simulink model "MineModel"  (R2024b)
settings: Solver=FixedStepAuto  StartTime=0.0  StopTime=5  FixedStep=1  RelTol=1e-3
values from neighbouring files (symbols this model uses):
  discountRate = dataFixed(4)    [practicalassignment.m]
undefined symbols (not defined in the file or in its folder): initialMiningCost, miningCostInflationRate
settings Model: Creator=veeti  LastModifiedBy=veeti

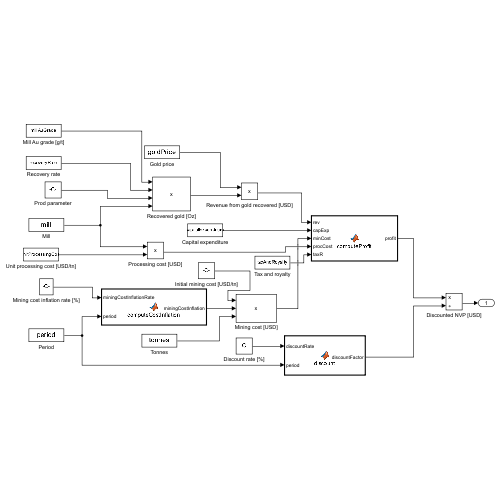
[thumbnail: Simulink's stored preview of the top-level diagram]
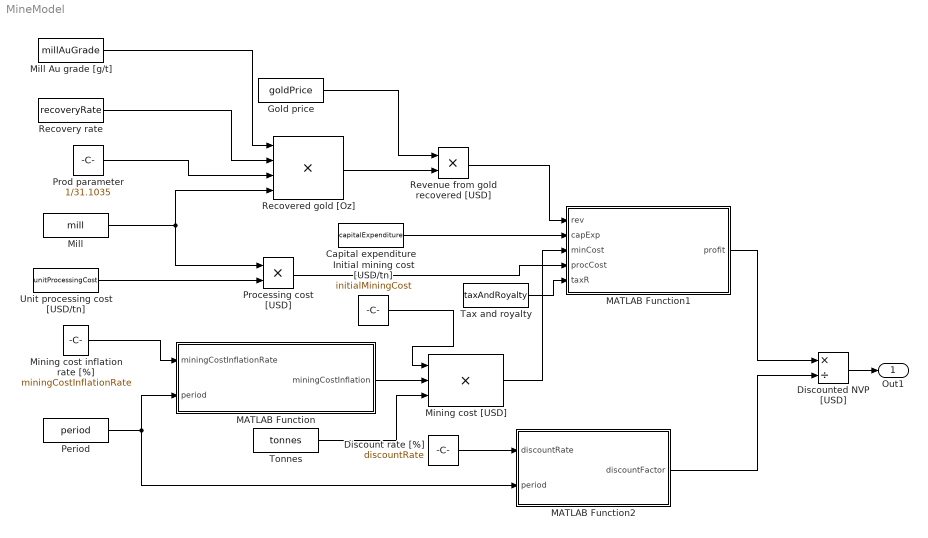
== system MineModel ==
  Capital expenditure : FromWorkspace  VariableName=capitalExpenditure
  Discount rate [%] : Constant  Value=discountRate
  Discounted NVP [USD] : Product  Inputs=*/
  Gold price : FromWorkspace  VariableName=goldPrice
  Initial mining cost [USD/tn] : Constant  Value=initialMiningCost
  MATLAB Function : MATLAB Function  TreatAsAtomicUnit=on
  MATLAB Function1 : MATLAB Function  TreatAsAtomicUnit=on
  MATLAB Function2 : MATLAB Function  TreatAsAtomicUnit=on
  Mill : FromWorkspace  VariableName=mill
  Mill Au grade [g/t] : FromWorkspace  VariableName=millAuGrade
  Mining cost [USD] : Product  Inputs=3
  Mining cost inflation rate [%] : Constant  Value=miningCostInflationRate
  Period : FromWorkspace  VariableName=period
  Processing cost [USD] : Product
  Prod parameter : Constant  Value=1/31.1035
  Recovered gold [Oz] : Product  Inputs=4
  Recovery rate : FromWorkspace  VariableName=recoveryRate
  Revenue from gold recovered [USD] : Product
  Tax and royalty : FromWorkspace  VariableName=taxAndRoyalty
  Tonnes : FromWorkspace  VariableName=tonnes
  Unit processing cost [USD/tn] : FromWorkspace  VariableName=unitProcessingCost
  Out1 : Outport
  wires:
  Mill/1 -> Recovered gold [Oz]/4, Processing cost [USD]/1
  Mill Au grade [g/t]/1 -> Recovered gold [Oz]/1
  Recovery rate/1 -> Recovered gold [Oz]/2
  Prod parameter/1 -> Recovered gold [Oz]/3
  Unit processing cost [USD/tn]/1 -> Processing cost [USD]/2
  Period/1 -> MATLAB Function2/2(period), MATLAB Function/2(period)
  Initial mining cost [USD/tn]/1 -> Mining cost [USD]/1
  MATLAB Function/1(miningCostInflation) -> Mining cost [USD]/2
  Tonnes/1 -> Mining cost [USD]/3
  Recovered gold [Oz]/1 -> Revenue from gold recovered [USD]/2
  Gold price/1 -> Revenue from gold recovered [USD]/1
  Revenue from gold recovered [USD]/1 -> MATLAB Function1/1(rev)
  Capital expenditure/1 -> MATLAB Function1/2(capExp)
  Mining cost [USD]/1 -> MATLAB Function1/3(minCost)
  Processing cost [USD]/1 -> MATLAB Function1/4(procCost)
  Tax and royalty/1 -> MATLAB Function1/5(taxR)
  Mining cost inflation rate [%]/1 -> MATLAB Function/1(miningCostInflationRate)
  Discount rate [%]/1 -> MATLAB Function2/1(discountRate)
  MATLAB Function1/1(profit) -> Discounted NVP [USD]/1
  MATLAB Function2/1(discountFactor) -> Discounted NVP [USD]/2
  Discounted NVP [USD]/1 -> Out1/1

== matlab function MineModel/MATLAB Function1 ==
  data: rev input; profit output; capExp input; minCost input; procCost input; taxR input
function profit = computeProfit(rev, capExp, minCost, procCost, taxR)
    profit = (rev-capExp-minCost-procCost)*(1-taxR);
end

== matlab function MineModel/MATLAB Function ==
  data: miningCostInflationRate input; miningCostInflation output; period input
function miningCostInflation = computeCostInflation(miningCostInflationRate, period)
miningCostInflation = (1+miningCostInflationRate/100)^(period-1);
end

== matlab function MineModel/MATLAB Function2 ==
  data: discountRate input; discountFactor output; period input
function discountFactor = discount(discountRate, period)
    discountFactor = (1+discountRate/100)^(period-1);
end
